simulink model "bench_motor"  (R2024b)
settings: Solver=daessc  StartTime=0.0  StopTime=20  MaxStep=1e-2  RelTol=1e-3
values from neighbouring files (symbols this model uses):
  PN = evalin('base','PN')    [run_bench_string_heat.m]
libraries: fl_lib x6, nesl_utility x4, sdl_lib x1, loco_native_lib x1
settings Model: Creator=BillBeverley  LastModifiedBy=BillBeverley

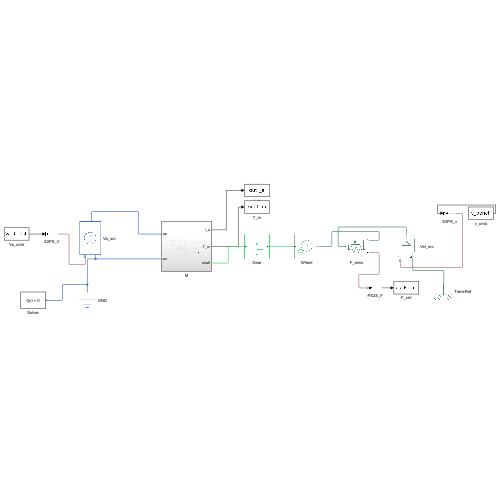
[thumbnail: Simulink's stored preview of the top-level diagram]
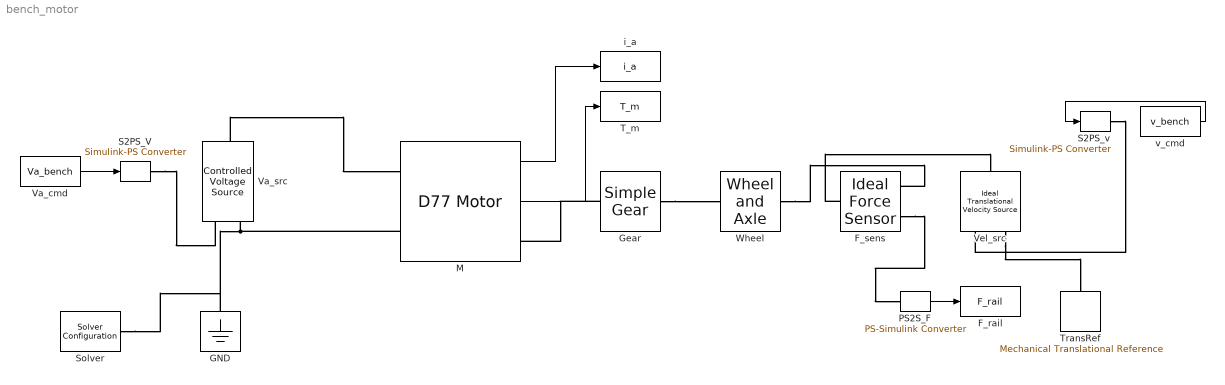
== system bench_motor ==
  F_rail : ToWorkspace  VariableName=F_rail  SaveFormat=Timeseries  SampleTime=-1
  F_sens : fl_lib/Mechanical/Mechanical Sensors/Ideal Force Sensor
  GND : fl_lib/Electrical/Electrical Elements/Electrical Reference
  Gear : sdl_lib/Gears/Simple Gear  ratio=PN.ax.G  rotation_direction=sdl.enum.shaftOutputDirection.same  friction_model=sdl.enum.gear_efficiencies_load.constant  T_noload=0.1 N*m  T_nom=5 N*m  efficiency_nom=0.8  efficiency=PN.ax.eta_g  temperature_TLU=[280, 300, 320] K  load_TLU=[1, 5, 10] N*m  efficiency_TLU=[.95, .9, .85]  efficiency_TLU2=[.85, .8, .75; .95, .9, .85; .85, .8, .7]  w_thr=0.01 rad/s  pwr_thr=1e3 W  enable_backlash=false  hardstop_model=simscape.enum.hardstop.smooth  backlash_distance=1e-3 mm  r_base=0.1 m  transition=1e-4 mm  backlash_stiffness=1e6 N/m  backlash_damping=1e3 N*s/m  coeff_rest=0.7  v_tol=0.001 m/s  f_tol=0.001 N  mu_visc=[0, 0] N*m*s/rad  thermal_mass=50 J/K  temperature_specify=off  temperature_priority=High  temperature=300 K  temperature_nominal_specify=off  temperature_nominal_value=1  temperature_nominal_unit=K  x_backlash_specify=off  x_backlash_priority=None  x_backlash=0 mm  x_backlash_nominal_specify=off  x_backlash_nominal_value=1  x_backlash_nominal_unit=mm  f_hardstop_specify=off  f_hardstop_priority=None  f_hardstop=0 N  f_hardstop_nominal_specify=off  f_hardstop_nominal_value=1  f_hardstop_nominal_unit=N  v_backlash_specify=off  v_backlash_priority=None  v_backlash=0 m/s  v_backlash_nominal_specify=off  v_backlash_nominal_value=1  v_backlash_nominal_unit=m/s
  M : loco_native_lib/D77 Motor  SystemSampleTime=-1  VariantActivationTime=update diagram  AllowFlexibleInterface=on  Latency=0  AutoFrameSizeCalculation=off
  PS2S_F : nesl_utility/PS-Simulink Converter  PhysicalDomain=network_engine_domain  SubClassName=ps_output  LeftPortType=input  RightPortType=output  PseudoPeriodic=off  Frequencies=[]  VectorFormat=inherit  Unit=N  AffineConversion=off
  S2PS_V : nesl_utility/Simulink-PS Converter  PhysicalDomain=network_engine_domain  SubClassName=ps_input  LeftPortType=input  RightPortType=output  PseudoPeriodic=off  Frequencies=[]  NoiseDistribution=none  NoiseParameters=[]  Unit=V  AffineConversion=off  FilteringAndDerivatives=provide  SimscapeFilterOrder=1  InputFilterTimeConstant=0.001  UdotUserProvided=0
  S2PS_v : nesl_utility/Simulink-PS Converter  PhysicalDomain=network_engine_domain  SubClassName=ps_input  LeftPortType=input  RightPortType=output  PseudoPeriodic=off  Frequencies=[]  NoiseDistribution=none  NoiseParameters=[]  Unit=m/s  AffineConversion=off  FilteringAndDerivatives=filter  SimscapeFilterOrder=1  InputFilterTimeConstant=0.001  UdotUserProvided=0
  Solver : nesl_utility/Solver Configuration  PhysicalDomain=network_engine_domain  SubClassName=solver  LeftPortType=input  RightPortType=generic  Tones=[]  Harmonics=[]  SimulateNoise=off  Profile=off  UseLocalSampling=off  EnableSwitchedLinearOptims=on  FrequencyDomain=off  UseCCode=off  RelTol=0.001  AbsTol=0.001  MinStep=1e-09  ToWorkspace=off  RevertToSquareIcSolve=off  NumHomotopyIterations=100  PhasorMode=off  PhasorModeNumHarmonics=1  ConsistencySolver=NEWTON_XTOL_AFTER_FTOL  IndexReductionMethod=DerivativeReplacement  DoDC=off  ResidualTolerance=1e-09  ConsistencyTolSource=GLOBAL  ConsistencyAbsTol=0.001  ConsistencyRelTol=0.001  ConsistencyTolFactor=0.001  UseLocalSolver=off  LocalSolverChoice=NE_BACKWARD_EULER_ADVANCER  ResolveIndetEquations=on  FunctionEvalNumThread=1  LocalSolverSampleTime=0.001  DoFixedCost=off  MaxNonlinIter=3  MaxModeIter=2  ComputeImpulses=off  ImpulseIterations=2  LinearAlgebra=auto  LinearAlgebraNumThread=0  EquationFormulation=NE_TIME_EF  DelaysMemoryBudget=1024  AutomaticFiltering=on  FilteringTimeConstant=0.001  PartitionStorageMethod=AS_NEEDED  PartitionMemoryBudget=1024  PartitionMethod=ROBUST  MultibodyUseLocalSolver=off  MultibodyLocalSolverChoice=ODE1  MultibodyLocalSolverSampleTime=0.001
  T_m : ToWorkspace  VariableName=T_m  SaveFormat=Timeseries  SampleTime=-1
  TransRef : fl_lib/Mechanical/Translational Elements/Mechanical Translational Reference
  Va_cmd : FromWorkspace  VariableName=Va_bench
  Va_src : fl_lib/Electrical/Electrical Sources/Controlled Voltage Source
  Vel_src : fl_lib/Mechanical/Mechanical Sources/Ideal Translational Velocity Source
  Wheel : fl_lib/Mechanical/Mechanisms/Wheel and Axle  R=PN.ax.r_w m  or=1  t_specify=off  t_priority=None  t=0 N*m  t_nominal_specify=off  t_nominal_value=1  t_nominal_unit=N*m  f_specify=off  f_priority=None  f=0 N  f_nominal_specify=off  f_nominal_value=1  f_nominal_unit=N
  i_a : ToWorkspace  VariableName=i_a  SaveFormat=Timeseries  SampleTime=-1
  v_cmd : FromWorkspace  VariableName=v_bench
  wires:
  Va_cmd/1 -> S2PS_V/1
  v_cmd/1 -> S2PS_v/1
  M/1 -> i_a/1
  M/2 -> T_m/1
  PS2S_F/1 -> F_rail/1
  connections:
  Va_src/LConn1 -- M/LConn1
  M/LConn2 -- Solver/RConn1 -- GND/LConn1 -- Va_src/RConn2
  S2PS_V/RConn1 -- Va_src/RConn1
  Gear/LConn1 -- M/RConn1
  Gear/RConn1 -- Wheel/LConn1
  Wheel/RConn1 -- F_sens/RConn1
  F_sens/LConn1 -- Vel_src/LConn1
  Vel_src/RConn2 -- TransRef/LConn1
  S2PS_v/RConn1 -- Vel_src/RConn1
  F_sens/RConn2 -- PS2S_F/LConn1
